simulink model "Acquisition"  (Simulink 8.9)
settings: Solver=VariableStepAuto  StartTime=0.0  StopTime=0.001  RelTol=1e-3
undefined symbols (not defined in the file or in its folder): get, Radix
libraries: dspxfrm3 x3, commsequence2 x1, simulink x1, dspsnks4 x1
settings Model: Creator=Alam  LastModifiedBy=Alam
settings SolverCC: AutoInsertRateTranBlk=on
settings DataIOCC: SaveFormat=Dataset  SignalLoggingSaveFormat=Dataset  SaveOutput=off  SignalLogging=off  SaveTime=off
settings DebuggingCC: AlgebraicLoopMsg=error  UnderspecifiedInitializationDetection=Simplified  MergeDetectMultiDrivingBlocksExec=error  SingleTaskRateTransMsg=error  FcnCallInpInsideContextMsg=error  AllowSymbolicDim=off  StateNameClashWarn=none
settings HardwareCC: ProdBitPerPointer=64  ProdBitPerSizeT=64  ProdBitPerPtrDiffT=64  ProdLargestAtomicFloat=Float  ProdIntDivRoundTo=Zero  ProdEndianess=LittleEndian  ProdWordSize=64  ProdHWDeviceType=Intel->x86-64 (Windows64)
settings ModelReferenceCC: PropagateSignalLabelsOutOfModel=on
settings GRTTargetCC: CombineOutputUpdateFcns=on  GRTInterface=off
settings ConfigComp: CovMetricSettings=dwe  CovHtmlReporting=off  CovSaveCumulativeToWorkspaceVar=off  CovSaveSingleToWorkspaceVar=off  CovExternalEMLEnable=on

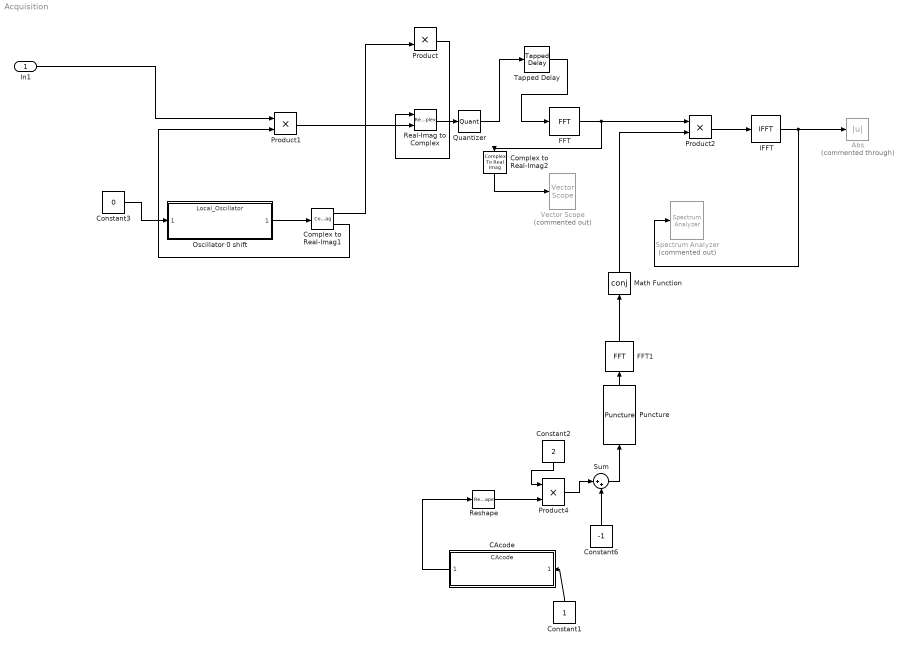
== system Acquisition ==
  In1 : Inport
  Abs : Abs  Commented=through
  CAcode : ModelReference  ModelNameDialog=CAcode.mdl  SimulationMode=Normal  ModelReferenceVersion=1.38
  Complex to Real-Imag1 : ComplexToRealImag
  Complex to Real-Imag2 : ComplexToRealImag  Output=Real
  Constant1 : Constant
  Constant2 : Constant  Value=2
  Constant3 : Constant  Value=0
  Constant6 : Constant  Value=-1
  FFT : dspxfrm3/FFT  FFTImplementation=Auto  CompMethod=Table lookup  TableOpt=NEW  TableOptActive=Speed  BitRevOrder=off  Normalize=off  InheritFFTLength=on  FFTLength=64  WrapInput=on  roundingMode=Floor  overflowMode=off  firstCoeffDataTypeStr=Inherit: Same word length as input  firstCoeffLastDataTypeStr=Inherit: Same word length as input  outputMin=[]  outputMax=[]
  FFT1 : dspxfrm3/FFT  FFTImplementation=Radix-2  CompMethod=Table lookup  TableOpt=NEW  TableOptActive=Speed  BitRevOrder=off  Normalize=off  InheritFFTLength=on  FFTLength=64  WrapInput=on  roundingMode=Floor  overflowMode=off  firstCoeffDataTypeStr=Inherit: Same word length as input  firstCoeffLastDataTypeStr=Inherit: Same word length as input  outputMin=[]  outputMax=[]
  IFFT : dspxfrm3/IFFT  FFTImplementation=Auto  CompMethod=Table lookup  TableOpt=NEW  TableOptActive=Speed  BitRevOrder=off  cs_in=off  Normalize=on  InheritFFTLength=on  FFTLength=64  WrapInput=on  mode=Complex  outSamplingMode=Sample based  roundingMode=Floor  overflowMode=off  firstCoeffDataTypeStr=Inherit: Same word length as input  firstCoeffLastDataTypeStr=Inherit: Same word length as input  outputMin=[]  outputMax=[]
      settings: SourceProductName=DSP System Toolbox
  Math Function : Math  Operator=conj  SaturateOnIntegerOverflow=on
  Oscillator 0 shift : ModelReference  ModelNameDialog=Local_Oscillator.slx  SimulationMode=Normal  ModelReferenceVersion=1.27
  Product{,1..2,4} (4 alike) : Product
  Puncture : commsequence2/Puncture  punctureVector=[1;0]
      settings: SourceProductName=Communications System Toolbox  SourceProductBaseCode=CM
  Quantizer : Quantizer
  Real-Imag to Complex : RealImagToComplex
  Reshape : Reshape  OutputDimensionality=Column vector (2-D)
  Spectrum Analyzer : SpectrumAnalyzer  Commented=on
  Sum : Sum  Inputs=|++
  Tapped Delay : simulink/Discrete/Tapped Delay  vinit=0.0  samptime=3.05175781e-8  NumDelays=32768  DelayOrder=Oldest  includeCurrent=off
  Vector Scope : dspsnks4/Vector Scope  Commented=on  ScopeProperties=on  Domain=Time  HorizSpan=1  DisplayProperties=off  AxisGrid=on  Memory=off  FrameNumber=on  AxisLegend=off  AxisZoom=off  OpenScopeAtSimStart=on  OpenScopeImmediately=off  FigPos=get(0,'defaultfigureposition')  AxisProperties=off  XUnits=Hertz  XRange=[0...Fs/2]  InheritXIncr=on  XIncr=1  XLabel=Time  XLimit=Auto  XMin=0  XMax=1  XStart=0  YUnits=dB  YLabel=Amplitude  LineProperties=off  XAxisParamsVer=6.9
      settings: SourceProductName=DSP System Toolbox  SourceProductBaseCode=DS  YMin=-10  YMax=10
  wires:
  FFT1/1 -> Math Function/1
  IFFT/1 -> Spectrum Analyzer/1, Abs/1
  CAcode/1 -> Reshape/1
  In1/1 -> Product1/1
  Product/1 -> Real-Imag to Complex/1
  Product1/1 -> Real-Imag to Complex/2
  Product2/1 -> IFFT/1
  Puncture/1 -> FFT1/1
  Constant1/1 -> CAcode/1
  Product4/1 -> Sum/1
  Constant6/1 -> Sum/2
  Constant2/1 -> Product4/1
  Reshape/1 -> Product4/2
  Sum/1 -> Puncture/1
  Real-Imag to Complex/1 -> Quantizer/1
  Math Function/1 -> Product2/2
  Tapped Delay/1 -> FFT/1
  Oscillator 0 shift/1 -> Complex to Real-Imag1/1
  Complex to Real-Imag1/1 -> Product/2
  Complex to Real-Imag1/2 -> Product1/2
  Constant3/1 -> Oscillator 0 shift/1
  Quantizer/1 -> Tapped Delay/1
  FFT/1 -> Complex to Real-Imag2/1, Product2/1
  Complex to Real-Imag2/1 -> Vector Scope/1
